simulink library "sm_trackV_lib_chain_contact_s46r4"  (R2026a)
settings: Solver=VariableStepAuto
undefined symbols (not defined in the file): Excv, P1, P2, P3, P4
libraries: sm_trackV_lib_chain_contact_s46 x4
Description:
  | Copyright 2024-2026 The MathWorks, Inc.
settings Model: Creator=smiller  LastModifiedBy=smiller

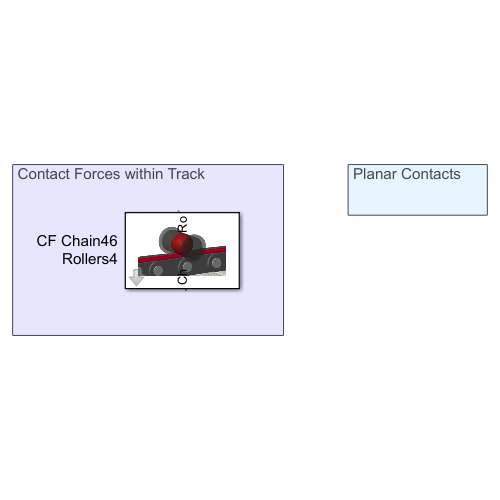
[thumbnail: Simulink's stored preview of the top-level diagram]
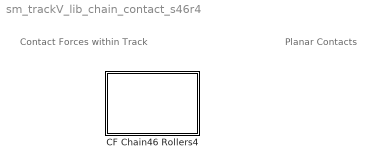
== system sm_trackV_lib_chain_contact_s46r4 ==
  note: Contact Forces within Track
  note: Planar Contacts
  CF Chain46 Rollers4 : Subsystem  mask(Contact Force, Full Chain to all Rollers){K_Roller=Excv.Contact.Roller.K, B_Roller=Excv.Contact.Roller.B, TW_Roller=Excv.Contact.Roller.TW}
      mask prompts: K_Roller "Normal Stiffness (N/m)"; B_Roller "Normal Damping (N/(m/s))"; TW_Roller "Normal Transition Width (m)"
      mask help: Models contact forces between entire chain and all rollers.
      mask Display: image('sm_excv_track_cf_chain_rollers_IMAGE.png')

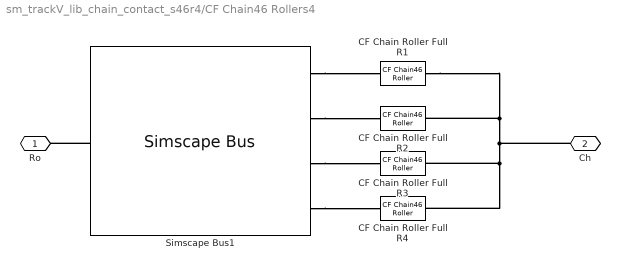
== system sm_trackV_lib_chain_contact_s46r4/CF Chain46 Rollers4 ==
  CF Chain Roller Full R{1..4} (4 alike) : sm_trackV_lib_chain_contact_s46/CF Chain46 Roller  K_Roller=K_Roller  B_Roller=B_Roller  TW_Roller=TW_Roller
  Simscape Bus1 : SimscapeBus  HierarchyStrings=P1;P2;P3;P4  ConnectionType=Bus: CBO_Roller4
  Ro : PMIOPort  Side=Left
  Ch : PMIOPort  Port=2  Side=Right
  connections:
  Simscape Bus1/RConn1 -- Ro/RConn1
  CF Chain Roller Full R3/RConn1 -- CF Chain Roller Full R1/RConn1 -- CF Chain Roller Full R2/RConn1 -- Ch/RConn1 -- CF Chain Roller Full R4/RConn1
  Simscape Bus1/LConn1 -- CF Chain Roller Full R1/LConn1
  Simscape Bus1/LConn2 -- CF Chain Roller Full R2/LConn1
  Simscape Bus1/LConn3 -- CF Chain Roller Full R3/LConn1
  Simscape Bus1/LConn4 -- CF Chain Roller Full R4/LConn1
